simulink model "lab6"  (R2022b)
settings: Solver=VariableStepAuto  StartTime=0.0  StopTime=10.0  RelTol=1e-3
undefined symbols (not defined in the file or in its folder): v
libraries: cstblocks x2
settings Model: Creator=S270874  LastModifiedBy=franc
settings ModelReferenceCC: EnableRefExpFcnMdlSchedulingChecks=on

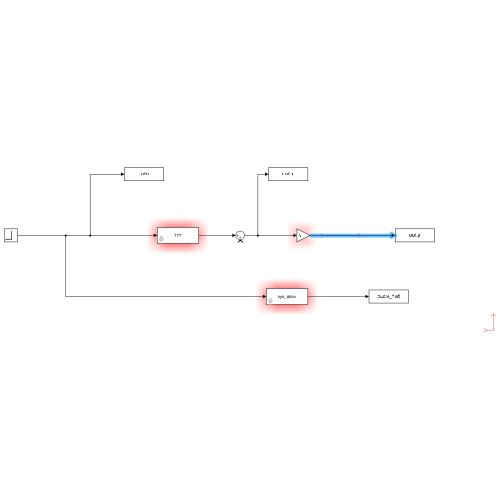
[thumbnail: Simulink's stored preview of the top-level diagram]
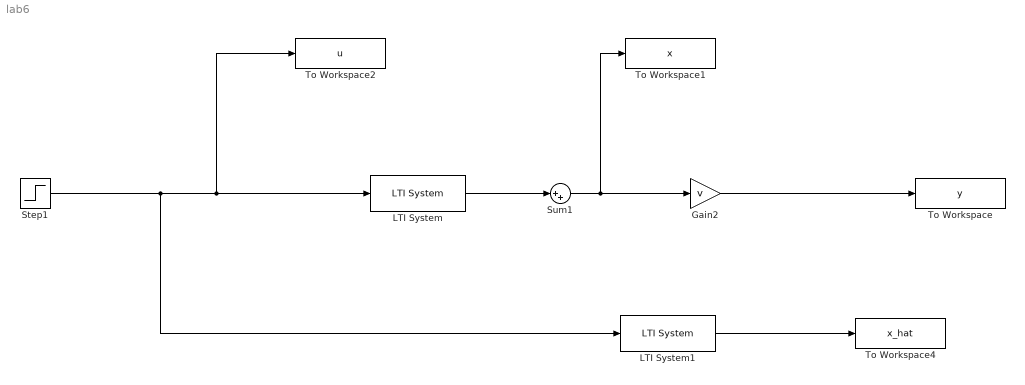
== system lab6 ==
  Gain2 : Gain  Gain=v
  LTI System : cstblocks/LTI System  sys=sys_x  IC=[]
  LTI System1 : cstblocks/LTI System  sys=sys_obsv  IC=[]
  Step1 : Step  Time=0  SampleTime=0
  Sum1 : Sum  Inputs=|++
  To Workspace : ToWorkspace  VariableName=y  SaveFormat=Timeseries  SampleTime=-1
  To Workspace1 : ToWorkspace  VariableName=x  SaveFormat=Timeseries  SampleTime=-1
  To Workspace2 : ToWorkspace  VariableName=u  SaveFormat=Timeseries  SampleTime=-1
  To Workspace4 : ToWorkspace  VariableName=x_hat  SaveFormat=Timeseries  SampleTime=-1
  wires:
  ? -> ?
  Sum1/1 -> Gain2/1, To Workspace1/1
  LTI System/1 -> Sum1/1
  ? -> ?
  Gain2/1 -> To Workspace/1
  Step1/1 -> LTI System1/1, To Workspace2/1, LTI System/1
  LTI System1/1 -> To Workspace4/1
